simulink model "VehicleDynamics"  (R2022a)
settings: Solver=VariableStepAuto  StartTime=0.0  StopTime=20  FixedStep=dt_sim  RelTol=1e-3  EnableMultiTasking=on
values from neighbouring files (symbols this model uses):
  A_sim = [(-CF-CR)/(m*Vv),(-CF*a+CR*b-m*Vv^2)/(m*Vv^2) ... (first row only)    [VehicleDynamics_init.m]    (also in s_track_ini.m)
  ay_max = 8    [VehicleDynamics_init.m]    (also in s_track_ini.m)
  B_sim = [CF/(m*Vv) CR/(m*Vv) ... (first row only)    [VehicleDynamics_init.m]    (also in s_track_ini.m)
  beta_max = 10    [VehicleDynamics_init.m]    (also in s_track_ini.m)
  C_sim = [1,0 ... (first row only)    [VehicleDynamics_init.m]    (also in s_track_ini.m)
  D_sim = [0 0 ... (first row only)    [VehicleDynamics_init.m]    (also in s_track_ini.m)
  delta_vol_max_ramp = 200    [VehicleDynamics_init.m]    (also in s_track_ini.m)
  dvol_max = 10    [VehicleDynamics_init.m]    (also in s_track_ini.m)
  L = 2.85    [VehicleDynamics_init.m]    (also in s_track_ini.m)
  sel_man = 1    [VehicleDynamics_init.m]    (also in s_track_ini.m)
  t_end_sim = 5    [VehicleDynamics_init.m]    (also in s_track_ini.m)
  tau_s = 15    [VehicleDynamics_init.m]    (also in s_track_ini.m)
  V = V/3.6    (= 27.7777777778)    [VehicleDynamics_init.m]    (also in s_track_ini.m)
libraries: simulink_extras x6, simulink x5, drivingvehiclecontroller x1
settings Model: Creator=gianl  LastModifiedBy=Vincentiu_Mocanu
settings SolverCC: AlgebraicLoopSolver=TrustRegion
settings DataIOCC: ReturnWorkspaceOutputs=off  ReturnWorkspaceOutputsName=out_SLX
settings OptimizationCC: LifeSpan=1
settings DebuggingCC: UnconnectedInputMsg=warning  UnconnectedOutputMsg=warning  UnconnectedLineMsg=warning  SFExecutionAtInitializationDiag=none  SFMachineParentedDataDiag=warning  ArithmeticOperatorsInVariantConditions=warning
settings SFSimCC: SimUseLocalCustomCode=off  CustomCodeUndefinedFunction=UseInterfaceOnly
settings RTWCC: RTWUseLocalCustomCode=off  DLArmComputeVersion=19.05
settings CodeAppCC: StateflowObjectComments=on

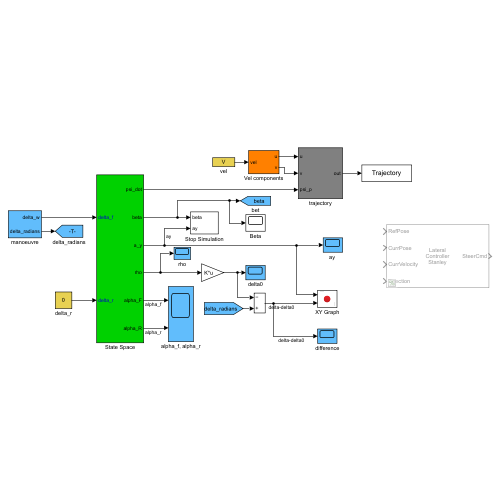
[thumbnail: Simulink's stored preview of the top-level diagram]
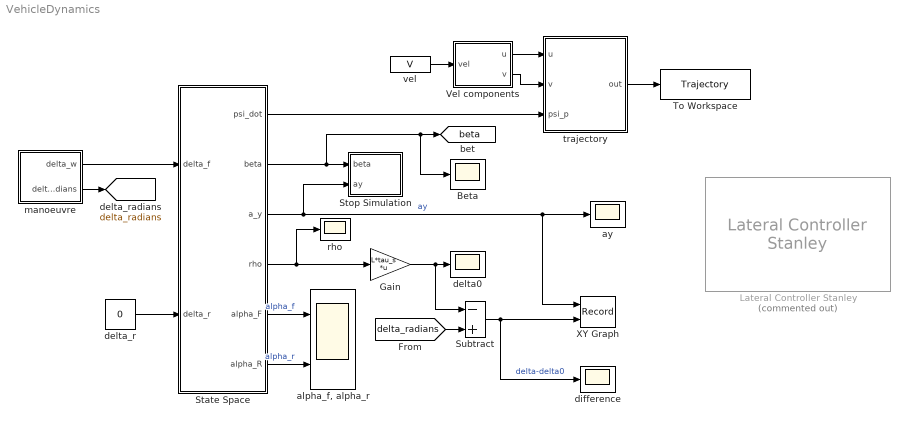
== system VehicleDynamics ==
  Beta : Scope
  Gain : Gain  Gain=L*tau_s  Multiplication=Matrix(K*u)
  Lateral Controller Stanley : drivingvehiclecontroller/Lateral Controller Stanley  Commented=on  ModelType=Kinematic bicycle model  PositionGainF=2.5  PositionGainR=2.5  YawRateGain=0.2  DelayGain=0.2  VehicleMass=1575  Lf=1.2  Lr=1.6  TireStiffness=19000  Wheelbase=2.8  MaxSteeringAngle=35
      settings: SourceProductBaseCode=DR
  State Space : Subsystem
  Stop Simulation : Subsystem
  Subtract : Sum  Inputs=-+
  To Workspace : ToWorkspace  VariableName=Trajectory  SaveFormat=Timeseries  SampleTime=-1
  Vel components : Subsystem
  XY Graph : Record  FileSettingsInternal="{\"entries\":[{\"content\":{\"excelSettings\":{\"content\":{},\"type\":\"Streamout.ExcelSettings\"}},\"type\":\"Streamout.FileSettingStorage\",\"uuid\":\"ca0bbbbb-2d8d-4106-81d8-32e5c71e5f3d\"}],\"packageUris\":[\"http://schema.mathworks.com/mf0/streamout_blocks/R2020a\"],\"version\":\"1.0\"}"  Layout=[1 1]  SignalsInternal="{\"entries\":[{\"content\":{\"signals\":[{\"content\":{\"blockPath\":[\"VehicleDynamics/XY Graph\"],\"channel\":[],\"dimensions\":[1],\"domain\":\"VehicleDynamics/XY Graph\",\"lineColor\":\"#a2142f\",\"plots\":[1],\"port\":1,\"sid\":[],\"signalID\":18,\"signalName\":\"ay\"},\"type\":\"RecordBlkView.Signal\",\"uuid\":\"a4082c68-e33f-4890-84c5-47a397f3ee8c\"},{\"content\":{\"blockPath\":[\"VehicleDynamics/XY Graph\"],\"channel\":[],\"dimensions\":[1],\"domain\":\"VehicleDynamics/XY Graph\",\"lineColor\":\"#139fff\",\"plots\":[1],\"port\":2,\"sid\":[],\"signalID\":21,\"signalName\":\"delta-delta0\"},\"type\":\"RecordBlkView.Signal\",\"uuid\":\"ec18cf13-4bd0-4e59-b066-a33baf30832d\"}]},\"type\":\"RecordBlkView.InputSignals\",\"uuid\":\"74c417fc-6621-41a2-9b06-b005b2f3cc1b\"}],\"packageUris\":[\"http://schema.mathworks.com/mf0/streamout_blocks/R2020a\"],\"version\":\"1.0\"}"  VisualizationBindings="{\"xyplotplugin\":{\"info\":[{\"series\":[{\"bindingParametersList\":[{\"parameter\":\"X-Axis\",\"signalID\":18,\"signalName\":\"ay\"},{\"parameter\":\"Y-Axis\",\"signalID\":21,\"signalName\":\"delta-delta0\"}],\"seriesID\":27305}],\"subplotID\":1}]}}"  CompatibilityTag=XY
  "alpha_f, alpha_r" : Scope  NumInputPorts=2
  "ay " : Scope
  delta0 : Scope
  delta_r : Constant  Value=0
  difference : Scope
  manoeuvre : Subsystem
  rho : Scope
  trajectory : Subsystem
  vel : Constant  Value=V
  tag scope: beta=global, delta_radians=global
  wires:
  manoeuvre/1(delta_w) -> State Space/1(delta_f)
  vel/1 -> Vel components/1(vel)
  Vel components/1(u) -> trajectory/1(u)
  Vel components/2(v) -> trajectory/2(v)
  delta_r/1 -> State Space/2(delta_r)
  State Space/5(alpha_F) -> "alpha_f, alpha_r"/1  "alpha_f"
  State Space/6(alpha_R) -> "alpha_f, alpha_r"/2  "alpha_r"
  State Space/4(rho) -> rho/1, Gain/1
  State Space/3(a_y) -> Stop Simulation/2(ay), XY Graph/1, "ay "/1  "ay"
  Gain/1 -> Subtract/1, delta0/1
  manoeuvre/2(delta_radians) -> [delta_radians]
  Subtract/1 -> difference/1, XY Graph/2  "delta-delta0"
  State Space/1(psi_dot) -> trajectory/3(psi_p)
  [delta_radians] -> Subtract/2
  State Space/2(beta) -> Beta/1, [beta], Stop Simulation/1(beta)
  trajectory/1(out) -> To Workspace/1

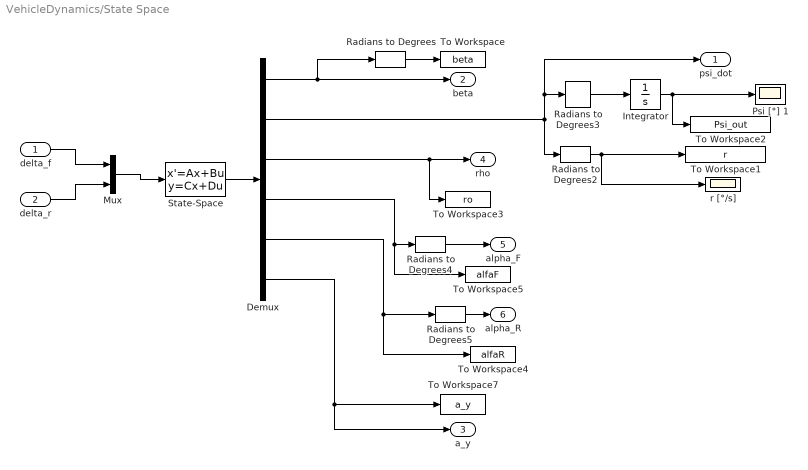
== system VehicleDynamics/State Space ==
  delta_f : Inport
  delta_r : Inport  Port=2
  Demux : Demux  Outputs=6
  Integrator : Integrator
  Mux : Mux  Inputs=2
  Psi [°] 1 : Scope
  Radians to Degrees{,2..5} (5 alike) : simulink_extras/Transformations/Radians to Degrees
  State-Space : StateSpace  A=A_sim  B=B_sim  C=C_sim  D=D_sim  InitialCondition=[0 0]  ContinuousStateAttributes={'sideslip_angle','yaw_rate'}
  To Workspace : ToWorkspace  VariableName=beta  SaveFormat=Timeseries  SampleTime=-1
  To Workspace1 : ToWorkspace  VariableName=r  SaveFormat=Timeseries  SampleTime=-1
  To Workspace2 : ToWorkspace  VariableName=Psi_out  SaveFormat=Timeseries  SampleTime=-1
  To Workspace3 : ToWorkspace  VariableName=ro  SaveFormat=Timeseries  SampleTime=-1
  To Workspace4 : ToWorkspace  VariableName=alfaR  SaveFormat=Timeseries  SampleTime=-1
  To Workspace5 : ToWorkspace  VariableName=alfaF  SaveFormat=Timeseries  SampleTime=-1
  To Workspace7 : ToWorkspace  VariableName=a_y  SaveFormat=Timeseries  SampleTime=-1
      settings: Save2DSignal=2-D array (concatenate along first dimension)
  r [°/s] : Scope
  psi_dot : Outport  VectorParamsAs1DForOutWhenUnconnected=off
  beta : Outport  Port=2  VectorParamsAs1DForOutWhenUnconnected=off
  a_y : Outport  Port=3  VectorParamsAs1DForOutWhenUnconnected=off
  rho : Outport  Port=4  VectorParamsAs1DForOutWhenUnconnected=off
  alpha_F : Outport  Port=5  VectorParamsAs1DForOutWhenUnconnected=off
  alpha_R : Outport  Port=6  VectorParamsAs1DForOutWhenUnconnected=off
  wires:
  Demux/2 -> psi_dot/1, Radians to Degrees3/1, Radians to Degrees2/1
  Demux/1 -> Radians to Degrees/1, beta/1
  State-Space/1 -> Demux/1
  Radians to Degrees/1 -> To Workspace/1
  Radians to Degrees2/1 -> r [°/s]/1, To Workspace1/1
  Demux/3 -> rho/1, To Workspace3/1
  Demux/4 -> Radians to Degrees4/1, To Workspace5/1
  Demux/5 -> Radians to Degrees5/1, To Workspace4/1
  Radians to Degrees3/1 -> Integrator/1
  Integrator/1 -> To Workspace2/1, Psi [°] 1/1
  delta_f/1 -> Mux/1
  Mux/1 -> State-Space/1
  delta_r/1 -> Mux/2
  Demux/6 -> a_y/1, To Workspace7/1
  Radians to Degrees4/1 -> alpha_F/1
  Radians to Degrees5/1 -> alpha_R/1

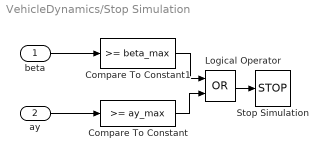
== system VehicleDynamics/Stop Simulation ==
  beta : Inport
  ay : Inport  Port=2
  Compare To Constant : simulink/Logic and Bit Operations/Compare To Constant  relop=>=  const=ay_max  OutDataTypeStr=boolean
  Compare To Constant1 : simulink/Logic and Bit Operations/Compare To Constant  relop=>=  const=beta_max  OutDataTypeStr=boolean
  Logical Operator : Logic  Operator=OR  AllPortsSameDT=off  OutDataTypeStr=boolean
  Stop Simulation : Stop
  wires:
  Logical Operator/1 -> Stop Simulation/1
  ay/1 -> Compare To Constant/1
  beta/1 -> Compare To Constant1/1
  Compare To Constant/1 -> Logical Operator/2
  Compare To Constant1/1 -> Logical Operator/1

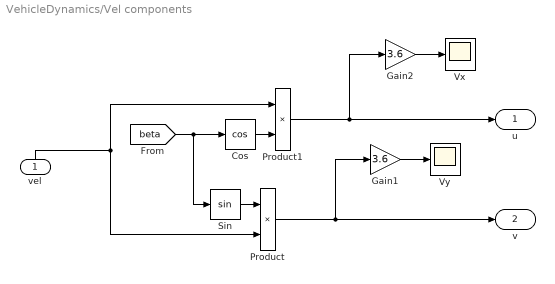
== system VehicleDynamics/Vel components ==
  vel : Inport
  Cos : Trigonometry  Operator=cos
  Gain1 : Gain  Gain=3.6
  Gain2 : Gain  Gain=3.6
  Product : Product
  Product1 : Product
  Sin : Trigonometry
  Vx : Scope
  Vy : Scope
  u : Outport  VectorParamsAs1DForOutWhenUnconnected=off
  v : Outport  Port=2  VectorParamsAs1DForOutWhenUnconnected=off
  wires:
  Product/1 -> Gain1/1, v/1
  Gain1/1 -> Vy/1
  Sin/1 -> Product/1
  Product1/1 -> u/1, Gain2/1
  vel/1 -> Product1/1, Product/2
  Gain2/1 -> Vx/1
  [beta] -> Sin/1, Cos/1
  Cos/1 -> Product1/2

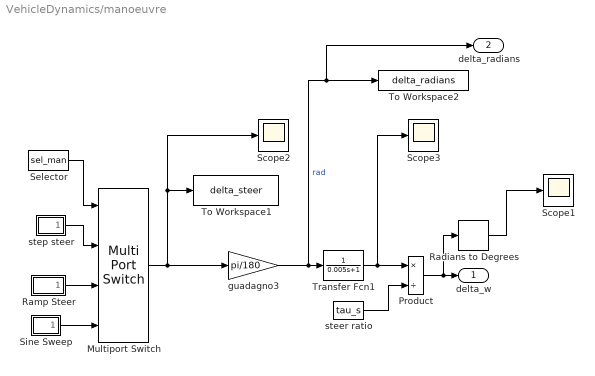
== system VehicleDynamics/manoeuvre ==
  Multiport Switch : MultiPortSwitch  SaturateOnIntegerOverflow=off  InputSameDT=off
  Product : Product  Inputs=*/  RndMeth=Zero
  Radians to Degrees : simulink_extras/Transformations/Radians to Degrees
  Ramp Steer : Subsystem
  Scope1 : Scope
  Scope2 : Scope
  Scope3 : Scope
  Selector : Constant  Value=sel_man
  Sine Sweep : Subsystem
  To Workspace1 : ToWorkspace  VariableName=delta_steer  SaveFormat=Timeseries  SampleTime=-1
  To Workspace2 : ToWorkspace  VariableName=delta_radians  SaveFormat=Timeseries  SampleTime=-1
  Transfer Fcn1 : TransferFcn  Denominator=[0.005 1]
  guadagno3 : Gain  Gain=pi/180  SaturateOnIntegerOverflow=on  OutDataTypeStr=Inherit: Same as input  ParamDataTypeStr=Inherit: Same as input
  "steer ratio " : Constant  Value=tau_s
  step steer : Subsystem
  delta_w : Outport  VectorParamsAs1DForOutWhenUnconnected=off
  delta_radians : Outport  Port=2  VectorParamsAs1DForOutWhenUnconnected=off
  wires:
  Selector/1 -> Multiport Switch/1
  Ramp Steer/1(delta) -> Multiport Switch/3
  step steer/1(delta) -> Multiport Switch/2
  Multiport Switch/1 -> To Workspace1/1, Scope2/1, guadagno3/1
  guadagno3/1 -> delta_radians/1, To Workspace2/1, Transfer Fcn1/1  "rad"
  "steer ratio "/1 -> Product/2
  Product/1 -> Radians to Degrees/1, delta_w/1
  Transfer Fcn1/1 -> Scope3/1, Product/1
  Radians to Degrees/1 -> Scope1/1
  Sine Sweep/1(delta) -> Multiport Switch/4

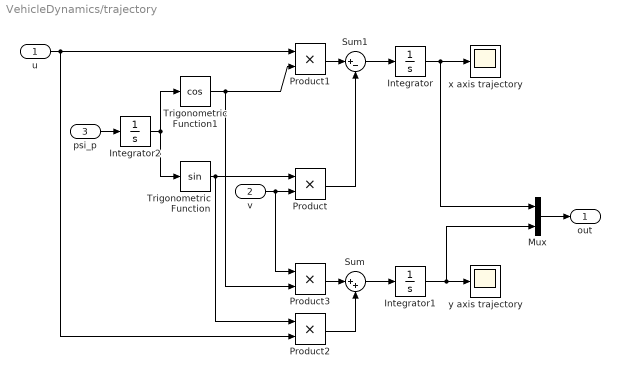
== system VehicleDynamics/trajectory ==
  u : Inport
  v : Inport  Port=2
  psi_p : Inport  Port=3
  Integrator : Integrator
  Integrator1 : Integrator
  Integrator2 : Integrator
  Mux : Mux  Inputs=2
  Product{,1..3} (4 alike) : Product  InputSameDT=on  SaturateOnIntegerOverflow=on  OutDataTypeStr=Inherit: Same as first input
  Sum : Sum  Inputs=|++  InputSameDT=on  SaturateOnIntegerOverflow=on  OutDataTypeStr=Inherit: Same as first input
  Sum1 : Sum  Inputs=|+-  InputSameDT=on  SaturateOnIntegerOverflow=on  OutDataTypeStr=Inherit: Same as first input
  Trigonometric Function : Trigonometry
  Trigonometric Function1 : Trigonometry  Operator=cos
  x axis trajectory : Scope
  y axis trajectory : Scope
  out : Outport
  wires:
  psi_p/1 -> Integrator2/1
  Product1/1 -> Sum1/1
  Product/1 -> Sum1/2
  Sum1/1 -> Integrator/1
  Trigonometric Function/1 -> Product/1, Product2/1
  u/1 -> Product2/2, Product1/1
  v/1 -> Product/2, Product3/1
  Trigonometric Function1/1 -> Product1/2, Product3/2
  Product3/1 -> Sum/1
  Product2/1 -> Sum/2
  Sum/1 -> Integrator1/1
  Integrator/1 -> Mux/1, x axis trajectory/1
  Integrator2/1 -> Trigonometric Function/1, Trigonometric Function1/1
  Integrator1/1 -> Mux/2, y axis trajectory/1
  Mux/1 -> out/1

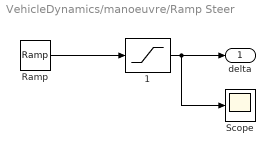
== system VehicleDynamics/manoeuvre/Ramp Steer ==
  "  1" : Saturate  UpperLimit=delta_vol_max_ramp  LowerLimit=-delta_vol_max_ramp
  Ramp : simulink/Sources/Ramp  slope=15  start=1  InitialOutput=0
  Scope : Scope
  delta : Outport  VectorParamsAs1DForOutWhenUnconnected=off
  wires:
  "  1"/1 -> Scope/1, delta/1
  Ramp/1 -> "  1"/1

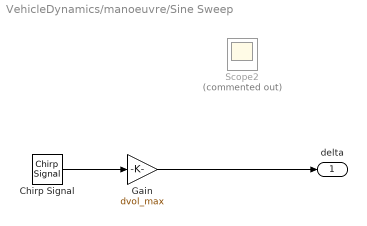
== system VehicleDynamics/manoeuvre/Sine Sweep ==
  Chirp Signal : simulink/Sources/Chirp Signal  f1=0.01  T=t_end_sim  f2=0.05
  Gain : Gain  Gain=dvol_max
  Scope2 : Scope  Commented=on
  delta : Outport  InitialOutput=0  VectorParamsAs1DForOutWhenUnconnected=off
  wires:
  Chirp Signal/1 -> Gain/1
  Gain/1 -> delta/1

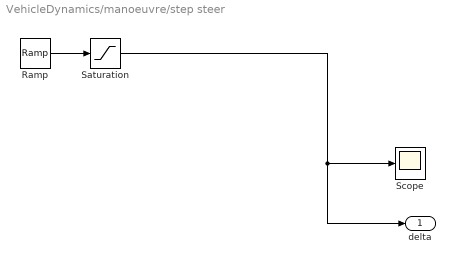
== system VehicleDynamics/manoeuvre/step steer ==
  Ramp : simulink/Sources/Ramp  slope=400  start=1  InitialOutput=0
  Saturation : Saturate  UpperLimit=dvol_max  LowerLimit=0
  Scope : Scope
  delta : Outport  VectorParamsAs1DForOutWhenUnconnected=off
  wires:
  Ramp/1 -> Saturation/1
  Saturation/1 -> delta/1, Scope/1
